simulink model "SubsystemTest2"  (R2020b)
settings: Solver=FixedStepAuto  StartTime=0.0  StopTime=48  FixedStep=0.1  RelTol=1e-3
settings Model: Creator=jim  LastModifiedBy=jim

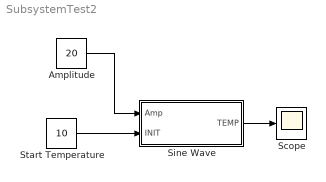
== system SubsystemTest2 ==
  Amplitude : Constant  Value=20
  Scope : Scope
  "Sine Wave " : Subsystem
  Start Temperature : Constant  Value=10
  wires:
  "Sine Wave "/1(TEMP) -> Scope/1
  Amplitude/1 -> "Sine Wave "/1(Amp)
  Start Temperature/1 -> "Sine Wave "/2(INIT)

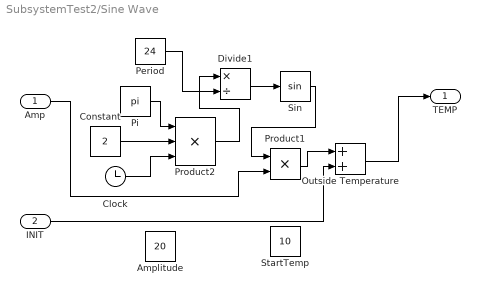
== system SubsystemTest2/Sine Wave  ==
  Amp : Inport
  INIT : Inport  Port=2
  Amplitude : Constant  Value=20
  Clock : Clock
  Constant : Constant  Value=2
  Divide1 : Product  Inputs=*/
  Outside Temperature : Sum
  Period : Constant  Value=24
  Pi : Constant  Value=pi  OutDataTypeStr=Inherit: Inherit via back propagation
  Product1 : Product
  Product2 : Product  Inputs=3
  Sin : Trigonometry
  StartTemp : Constant  Value=10
  TEMP : Outport
  wires:
  Divide1/1 -> Sin/1
  Product2/1 -> Divide1/1
  Constant/1 -> Product2/2
  Sin/1 -> Product1/1
  Pi/1 -> Product2/1
  Clock/1 -> Product2/3
  Period/1 -> Divide1/2
  Product1/1 -> Outside Temperature/1
  Outside Temperature/1 -> TEMP/1
  Amp/1 -> Product1/2
  INIT/1 -> Outside Temperature/2
